simulink model "testing_interpolation"  (R2022a)
settings: Solver=VariableStepAuto  StartTime=0.0  StopTime=0.3  RelTol=1e-3
libraries: SignalEditorBlockLib x1
settings Model: PacingRate=0.100000  Creator=gautamd  LastModifiedBy=gautamd

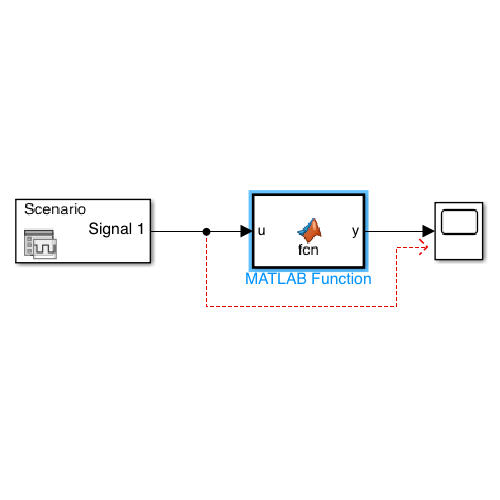
[thumbnail: Simulink's stored preview of the top-level diagram]
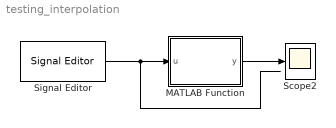
== system testing_interpolation ==
  MATLAB Function : MATLAB Function  TreatAsAtomicUnit=on
  Scope2 : Scope
  Signal Editor : SignalEditorBlockLib/Signal Editor  FileName=temp_distance_vs_time.mat  ActiveScenario=Scenario  ActiveSignal=Signal 1  IsBus=off  OutputBusObjectStr=Bus: BusObject  SampleTime=0  ZeroCross=off  OutputAfterFinalValue=Setting to zero  Unit=inherit  PreserveSignalName=on
  wires:
  MATLAB Function/1(y) -> Scope2/1
  Signal Editor/1 -> MATLAB Function/1(u)

== matlab function testing_interpolation/MATLAB Function ==
  data: u input; y output
function y = fcn(u)

tc = load("track.mat");

track_cumulative = tc.track_cumulative;

a = track_cumulative(:,3,:)./track_cumulative(:,1,:);
b = track_cumulative(:,4,:);

y = 1/interp1(b,a,u,"previous");
